simulink model "model_5"  (R2020a)
settings: Solver=VariableStepAuto  StartTime=0.0  StopTime=30  RelTol=1e-3
settings Model: Creator=Notnik_kg  LastModifiedBy=Notnik_kg

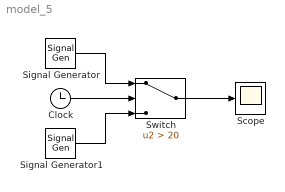
== system model_5 ==
  Clock : Clock
  Scope : Scope
  Signal Generator : SignalGenerator  WaveForm=sawtooth  Units=rad/sec
  Signal Generator1 : SignalGenerator  WaveForm=square  Units=rad/sec
  Switch : Switch  Criteria=u2 > Threshold  Threshold=20
  wires:
  Signal Generator/1 -> Switch/1
  Clock/1 -> Switch/2
  Signal Generator1/1 -> Switch/3
  Switch/1 -> Scope/1
